simulink model "horno_baja_temperatura"  (R2015a)
settings: Solver=ode45  StartTime=0.0  StopTime=1500  RelTol=1e-3
libraries: simulink x2
settings Model: Creator=m4v  LastModifiedBy=m4v

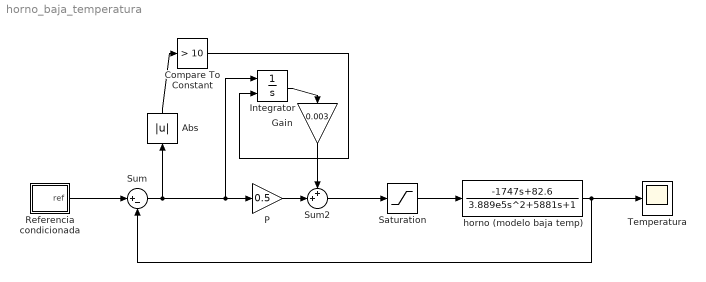
== system horno_baja_temperatura ==
  Abs : Abs
  Compare To Constant : simulink/Logic and Bit Operations/Compare To Constant  relop=>  const=10  OutDataTypeStr=boolean
  Gain : Gain  Gain=0.003
  Integrator : Integrator  ExternalReset=level
  P : Gain  Gain=0.5
  Referencia condicionada : Subsystem
  Saturation : Saturate  UpperLimit=100  LowerLimit=0  ZeroCross=off
  Sum : Sum  Inputs=|+-
  Sum2 : Sum  Inputs=++|
  Temperatura : Scope
      settings: TimeRange=1500  YMin=-50  YMax=250  SampleInput=on  SampleTime=1
  horno (modelo baja temp) : TransferFcn  Numerator=[-1747 82.6]  Denominator=[3.889e5 5881 1]
  wires:
  horno (modelo baja temp)/1 -> Sum/2, Temperatura/1
  Sum2/1 -> Saturation/1
  Saturation/1 -> horno (modelo baja temp)/1
  P/1 -> Sum2/2
  Integrator/1 -> Gain/1
  Gain/1 -> Sum2/1
  Abs/1 -> Compare To Constant/1
  Compare To Constant/1 -> Integrator/2
  Sum/1 -> Abs/1, P/1, Integrator/1
  Referencia condicionada/1(ref) -> Sum/1

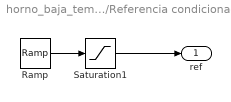
== system horno_baja_temperatura/Referencia condicionada ==
  Ramp : simulink/Sources/Ramp  slope=0.3333  start=0  X0=0
  Saturation1 : Saturate  UpperLimit=168.99  LowerLimit=0
  ref : Outport
  wires:
  Ramp/1 -> Saturation1/1
  Saturation1/1 -> ref/1
